simulink library "library_PX4SITLConnection"  (R2024a)
settings: Solver=VariableStepAuto  StartTime=0.0  StopTime=10.0  RelTol=1e-3
libraries: library_PX4SITLSFunc x1
settings Model: Creator=tommy  LastModifiedBy=tommy

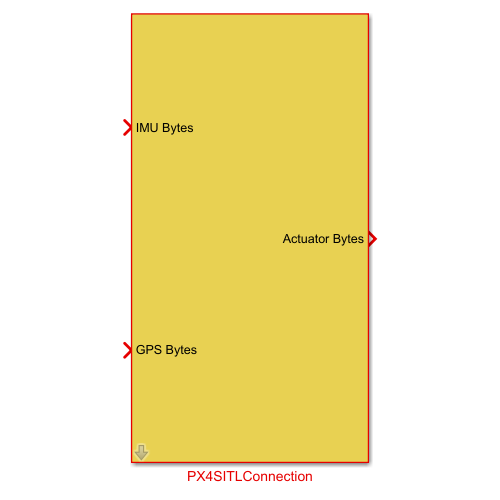
[thumbnail: Simulink's stored preview of the top-level diagram]
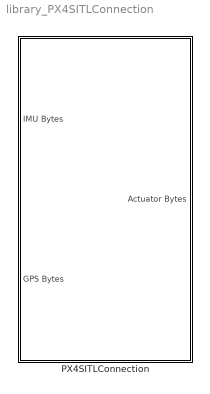
== system library_PX4SITLConnection ==
  PX4SITLConnection : Subsystem
      mask help: Default Mask

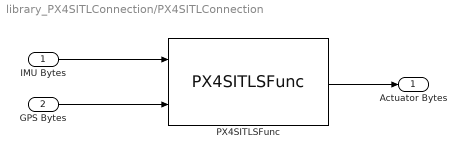
== system library_PX4SITLConnection/PX4SITLConnection ==
  IMU Bytes : Inport
  GPS Bytes : Inport  Port=2
  PX4SITLSFunc : library_PX4SITLSFunc/PX4SITLSFunc
  Actuator Bytes : Outport
  wires:
  IMU Bytes/1 -> PX4SITLSFunc/1
  GPS Bytes/1 -> PX4SITLSFunc/2
  PX4SITLSFunc/1 -> Actuator Bytes/1
